simulink model "BoatLibrary"  (Simulink 7.9)
settings: Solver=ode45  StartTime=0.0  StopTime=10.0  RelTol=1e-3
values from neighbouring files (symbols this model uses):
  C = C0    [Minimizer.m]    (also in parameters2.m = [1 0 0 0 0 0;0 0 1 0 0 0;0 0 0 0 1 0]; parameters3.m = [1 0 0 0 0 0;0 0 1 0 0 0;0 0 0 0 1 0])
  fw = 4    [parameters2.m]    (also in parameters3.m)
  I = 1/12*M*((2*rx1)^2 + (2*ry1)^2)    (= 7.46230507536)    [BoatController.m]    (also in boatDynamics.m; parameters2.m = 20; parameters3.m)
  K = [1000 1000 1000 10 10 1 1]    [parameters3.m]
  kr = 2    [parameters2.m]    (also in parameters3.m)
  M = 80*lbtokg    (= 36.28736)    [BoatController.m]    (also in parameters2.m = 10; parameters3.m)
  rx1 = -12*intom    (= -0.3048)    [BoatController.m]    (also in boatDynamics.m; costfunction.m; parameters3.m)
  rx2 = 12*intom    (= 0.3048)    [BoatController.m]    (also in boatDynamics.m; costfunction.m; parameters3.m)
  ry1 = -69*intom/2 + 6*intom    (= -0.7239)    [BoatController.m]    (also in boatDynamics.m; costfunction.m; parameters3.m)
  ry2 = ry1    (= -0.7239)    [BoatController.m]    (also in boatDynamics.m; costfunction.m; parameters3.m)
libraries: simulink x3
settings Model: Creator=Darsan  LastModifiedBy=Darsan

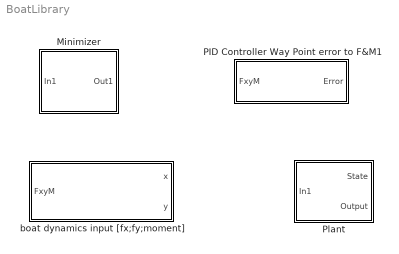
== system BoatLibrary ==
  Minimizer : Subsystem  mask{rx1=rx1, rx2=rx2, ry1=ry1, ry2=ry2, C=K}
      mask prompts: C "Performance Gain"
  PID Controller Way Point error to F&M1 : Subsystem
  Plant : Subsystem  mask{rx1=rx1, rx2=rx2, ry1=ry1, ry2=ry2, M=M, I=I, C=C}
  boat dynamics input [fx;fy;moment] : Subsystem  mask{M=M, I=I, fw=fw, kr=kr, C=C}
      mask prompts: M "Mass"; I "Inert"; fw "Water Friction"; kr "Rotational water Friction"; C "Output Matrix"

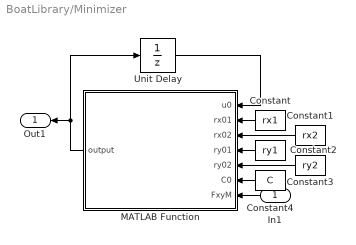
== system BoatLibrary/Minimizer ==
  In1 : Inport
  Constant : Constant  Value=rx1
  Constant1 : Constant  Value=rx2
  Constant2 : Constant  Value=ry1
  Constant3 : Constant  Value=ry2
  Constant4 : Constant  Value=C
  MATLAB Function : MATLAB Function  TreatAsAtomicUnit=on
  Unit Delay : UnitDelay  SampleTime=-1
  Out1 : Outport
  wires:
  In1/1 -> MATLAB Function/7(FxyM)
  MATLAB Function/1(output) -> Out1/1, Unit Delay/1
  Unit Delay/1 -> MATLAB Function/1(u0)
  Constant4/1 -> MATLAB Function/6(C0)
  Constant3/1 -> MATLAB Function/5(ry02)
  Constant2/1 -> MATLAB Function/4(ry01)
  Constant1/1 -> MATLAB Function/3(rx02)
  Constant/1 -> MATLAB Function/2(rx01)

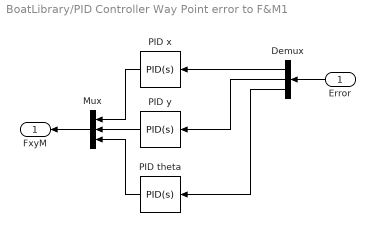
== system BoatLibrary/PID Controller Way Point error to F&M1 ==
  Error : Inport
  Demux : Demux  Outputs=3
  Mux : Mux  Inputs=3
  PID theta : simulink/Continuous/PID Controller  Controller=PID  TimeDomain=Continuous-time  SampleTime=1  IntegratorMethod=Forward Euler  FilterMethod=Forward Euler  Form=Parallel  P=-52.7411095906827  I=-178.448916818041  D=5.47077070641916  N=9.64052643054454  InitialConditionSource=internal  InitialConditionForIntegrator=0  InitialConditionForFilter=0  ExternalReset=none  LimitOutput=off  UpperSaturationLimit=inf  LowerSaturationLimit=-inf  LinearizeAsGain=off  AntiWindupMode=none  Kb=1  TrackingMode=off  Kt=1  PParamMin=[]  PParamMax=[]  IParamMin=[]  IParamMax=[]  DParamMin=[]  DParamMax=[]  NParamMin=[]  NParamMax=[]  KbParamMin=[]  KbParamMax=[]  KtParamMin=[]  KtParamMax=[]  POutMin=[]  POutMax=[]  IOutMin=[]  IOutMax=[]  DOutMin=[]  DOutMax=[]  NOutMin=[]  NOutMax=[]  KbOutMin=[]  KbOutMax=[]  KtOutMin=[]  KtOutMax=[]  IntegratorOutMin=[]  IntegratorOutMax=[]  FilterOutMin=[]  FilterOutMax=[]  SumOutMin=[]  SumOutMax=[]  SumI1OutMin=[]  SumI1OutMax=[]  SumI2OutMin=[]  SumI2OutMax=[]  SumI3OutMin=[]  SumI3OutMax=[]  SumDOutMin=[]  SumDOutMax=[]  SaturationOutMin=[]  SaturationOutMax=[]  IntegratorContinuousStateAttributes=''  IntegratorStateMustResolveToSignalObject=off  IntegratorRTWStateStorageClass=Auto  FilterContinuousStateAttributes=''  FilterStateMustResolveToSignalObject=off  FilterRTWStateStorageClass=Auto
  PID x : simulink/Continuous/PID Controller  Controller=PID  TimeDomain=Continuous-time  SampleTime=1  IntegratorMethod=Forward Euler  FilterMethod=Forward Euler  Form=Parallel  P=-52.7411095906827  I=-356.897833636081  D=2.73538535320958  N=19.2810528610891  InitialConditionSource=internal  InitialConditionForIntegrator=0  InitialConditionForFilter=0  ExternalReset=none  LimitOutput=off  UpperSaturationLimit=inf  LowerSaturationLimit=-inf  LinearizeAsGain=off  AntiWindupMode=none  Kb=1  TrackingMode=off  Kt=1  PParamMin=[]  PParamMax=[]  IParamMin=[]  IParamMax=[]  DParamMin=[]  DParamMax=[]  NParamMin=[]  NParamMax=[]  KbParamMin=[]  KbParamMax=[]  KtParamMin=[]  KtParamMax=[]  POutMin=[]  POutMax=[]  IOutMin=[]  IOutMax=[]  DOutMin=[]  DOutMax=[]  NOutMin=[]  NOutMax=[]  KbOutMin=[]  KbOutMax=[]  KtOutMin=[]  KtOutMax=[]  IntegratorOutMin=[]  IntegratorOutMax=[]  FilterOutMin=[]  FilterOutMax=[]  SumOutMin=[]  SumOutMax=[]  SumI1OutMin=[]  SumI1OutMax=[]  SumI2OutMin=[]  SumI2OutMax=[]  SumI3OutMin=[]  SumI3OutMax=[]  SumDOutMin=[]  SumDOutMax=[]  SaturationOutMin=[]  SaturationOutMax=[]  IntegratorContinuousStateAttributes=''  IntegratorStateMustResolveToSignalObject=off  IntegratorRTWStateStorageClass=Auto  FilterContinuousStateAttributes=''  FilterStateMustResolveToSignalObject=off  FilterRTWStateStorageClass=Auto
  PID y : simulink/Continuous/PID Controller  Controller=PID  TimeDomain=Continuous-time  SampleTime=1  IntegratorMethod=Forward Euler  FilterMethod=Forward Euler  Form=Parallel  P=-52.7411095906827  I=-356.897833636081  D=2.73538535320958  N=19.2810528610891  InitialConditionSource=internal  InitialConditionForIntegrator=0  InitialConditionForFilter=0  ExternalReset=none  LimitOutput=off  UpperSaturationLimit=inf  LowerSaturationLimit=-inf  LinearizeAsGain=off  AntiWindupMode=none  Kb=1  TrackingMode=off  Kt=1  PParamMin=[]  PParamMax=[]  IParamMin=[]  IParamMax=[]  DParamMin=[]  DParamMax=[]  NParamMin=[]  NParamMax=[]  KbParamMin=[]  KbParamMax=[]  KtParamMin=[]  KtParamMax=[]  POutMin=[]  POutMax=[]  IOutMin=[]  IOutMax=[]  DOutMin=[]  DOutMax=[]  NOutMin=[]  NOutMax=[]  KbOutMin=[]  KbOutMax=[]  KtOutMin=[]  KtOutMax=[]  IntegratorOutMin=[]  IntegratorOutMax=[]  FilterOutMin=[]  FilterOutMax=[]  SumOutMin=[]  SumOutMax=[]  SumI1OutMin=[]  SumI1OutMax=[]  SumI2OutMin=[]  SumI2OutMax=[]  SumI3OutMin=[]  SumI3OutMax=[]  SumDOutMin=[]  SumDOutMax=[]  SaturationOutMin=[]  SaturationOutMax=[]  IntegratorContinuousStateAttributes=''  IntegratorStateMustResolveToSignalObject=off  IntegratorRTWStateStorageClass=Auto  FilterContinuousStateAttributes=''  FilterStateMustResolveToSignalObject=off  FilterRTWStateStorageClass=Auto
  FxyM : Outport
  wires:
  Mux/1 -> FxyM/1
  PID theta/1 -> Mux/3
  PID x/1 -> Mux/1
  PID y/1 -> Mux/2
  Error/1 -> Demux/1
  Demux/3 -> PID theta/1
  Demux/2 -> PID y/1
  Demux/1 -> PID x/1

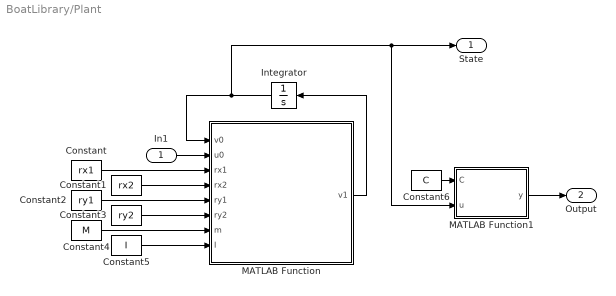
== system BoatLibrary/Plant ==
  In1 : Inport
  Constant : Constant  Value=rx1
  Constant1 : Constant  Value=rx2
  Constant2 : Constant  Value=ry1
  Constant3 : Constant  Value=ry2
  Constant4 : Constant  Value=M
  Constant5 : Constant  Value=I
  Constant6 : Constant  Value=C
  Integrator : Integrator  InitialCondition=[0 0 0 0 0 0]
  MATLAB Function : MATLAB Function  TreatAsAtomicUnit=on
  MATLAB Function1 : MATLAB Function  TreatAsAtomicUnit=on
  State : Outport
  Output : Outport  Port=2
  wires:
  MATLAB Function1/1(y) -> Output/1
  Constant6/1 -> MATLAB Function1/1(C)
  In1/1 -> MATLAB Function/2(u0)
  Integrator/1 -> MATLAB Function1/2(u), State/1, MATLAB Function/1(v0)
  MATLAB Function/1(v1) -> Integrator/1
  Constant5/1 -> MATLAB Function/8(I)
  Constant4/1 -> MATLAB Function/7(m)
  Constant3/1 -> MATLAB Function/6(ry2)
  Constant2/1 -> MATLAB Function/5(ry1)
  Constant1/1 -> MATLAB Function/4(rx2)
  Constant/1 -> MATLAB Function/3(rx1)

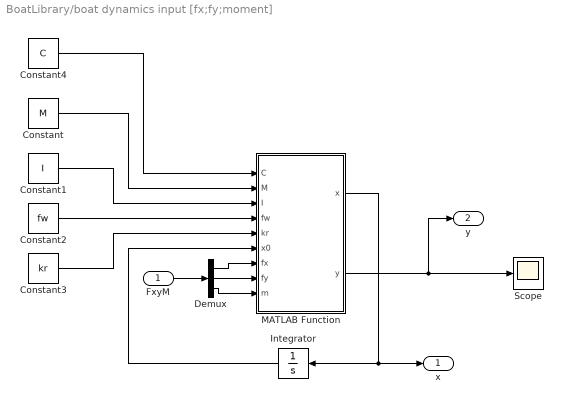
== system BoatLibrary/boat dynamics input [fx;fy;moment] ==
  FxyM : Inport
  Constant : Constant  Value=M
  Constant1 : Constant  Value=I
  Constant2 : Constant  Value=fw
  Constant3 : Constant  Value=kr
  Constant4 : Constant  Value=C
  Demux : Demux  Outputs=3
  Integrator : Integrator  InitialCondition=[0 0 0 0 0 0]
  MATLAB Function : MATLAB Function  TreatAsAtomicUnit=on
  Scope : Scope
  x : Outport
  y : Outport  Port=2
  wires:
  Demux/3 -> MATLAB Function/9(m)
  Demux/2 -> MATLAB Function/8(fy)
  Demux/1 -> MATLAB Function/7(fx)
  FxyM/1 -> Demux/1
  MATLAB Function/1(x) -> x/1, Integrator/1
  Constant4/1 -> MATLAB Function/1(C)
  Constant3/1 -> MATLAB Function/5(kr)
  Constant2/1 -> MATLAB Function/4(fw)
  Constant1/1 -> MATLAB Function/3(I)
  Constant/1 -> MATLAB Function/2(M)
  Integrator/1 -> MATLAB Function/6(x0)
  MATLAB Function/2(y) -> y/1, Scope/1

== matlab function Plant/MATLAB Function ==
  data: v0 input double; v1 output double; u0 input double; rx1 input double; rx2 input double; ry1 input double; ry2 input double; m input double; I input double
function v1   = boatDynamics(v0, u0, rx1, rx2, ry1, ry2, m, I)

    % %%%%%%%%%%%%%%%%%%%%%%%%%%%%%%%%%%%%%%%%%%%% %
    %    v = [x...          %    u = [theta1...    %
    %        x_dot...       %        f1...         %
    %        y...           %        theta2...     %
    %        y_dot...       %        f2]           %
    %        theta...       %                      %
    %        theta_dot];    %                      %
    % %%%%%%%%%%%%%%%%%%%%%%%%%%%%%%%%%%%%%%%%%%%% %
    
    v11 = v0(2);
    v12 = -u0(2)/m*sind(u0(1)+v0(5)) - u0(4)/m*sind(u0(3)+v0(5)) - 0*5*v0(1);
    v13 = v0(4);
    v14 = u0(2)/m*cosd(u0(1)+v0(5)) + u0(4)/m*cosd(u0(3)+v0(5)) - 0*2*v0(3);
    v15 = v0(6);
    v16 = rx1/I*u0(2)*cosd(u0(1)) + ry1/I*u0(2)*sind(u0(1)) + rx2/I*u0(4)*cosd(u0(3)) + ry2/I*u0(4)*sind(u0(3)) - 0*9*v0(5);
   
    v1 = [v11;v12;v13;v14;v15;v16];
    
    
end

== matlab function boat dynamics input [fx;fy;moment]/MATLAB Function ==
  data: C input double; x output double; M input double; I input double; fw input double; kr input double; x0 input double; fx input double; y output double; fy input double; m input double
function [x,y] = systemstep(C,M,I,fw,kr,x0,fx,fy,m)

   % status vector y=[x;x_dot;y;_y_dot;theta;theta_dot]
   % forces u=[fx;fy;m]
   % contant parameters {mass; rotational inertia; friction coefficients }
   
   x1 = x0(2);
   x2 = fx/M - x0(2)*fw;
   x3 = x0(4);
   x4 = fy/M - x0(4)*fw;
   x5 = x0(6);
   x6 = m/I - x0(6)*kr;

   x=[x1;x2;x3;x4;x5;x6];
   
   y = C*x;

== matlab function Minimizer/MATLAB Function ==
  data: u0 input double; output output double; rx01 input double; rx02 input double; ry01 input double; ry02 input double; C0 input double; FxyM input double
function output = Minimizer(u0, rx01, rx02, ry01, ry02, C0, FxyM)

% global rx1 rx2 ry1 ry2 C;
% global Fxref Fyref Mref;

rx1 = rx01; rx2 = rx02;
ry1 = ry01; ry2 = ry02;

C = C0;

Fxref = FxyM(1); Fyref = FxyM(2); Mref  = FxyM(3);
u1 = u0;

    for k = 1:3
        h = getDirection(u1, u0, Fxref, Fyref, Mref, rx1, rx2, ry1, ry2, C);
        alpha = getStepSize(u1, u0, h, Fxref, Fyref, Mref, rx1, rx2, ry1, ry2, C);
        u1 = u1 + alpha*h;
    end
    
    output = u1;

end

function output = getStepSize(input, preinput, h, Fxref, Fyref, Mref, rx1, rx2, ry1, ry2, C)

%     global Fxref Fyref Mref;

    alpha = 1;
    
    u0 = input;
    u1 = input + alpha*h;
    
    v0 = costFunction( u0, preinput, Fxref, Fyref, Mref, rx1, rx2, ry1, ry2, C );
    v1 = costFunction( u1, preinput, Fxref, Fyref, Mref, rx1, rx2, ry1, ry2, C );

    while v1 < v0
        alpha = alpha + 1;
        u1 = input + alpha*h;
        v0 = v1;
        v1 = costFunction( u1, preinput, Fxref, Fyref, Mref, rx1, rx2, ry1, ry2, C );
    end

    while v1 > v0 && alpha > 0
        alpha = alpha - 0.1;
        u1 = input + alpha*h;
        v0 = v1;
        v1 = costFunction( u1, preinput, Fxref, Fyref, Mref, rx1, rx2, ry1, ry2, C );
    end

    output = alpha;

end

function output = costFunction(input, preinput, Fxref, Fyref, Mref, rx1, rx2, ry1, ry2, C)

% global rx1 rx2 ry1 ry2 C;
% global Fxref Fyref Mref;

    theta1  = input(1);
    f1      = input(2);
    theta2  = input(3);
    f2      = input(4);
    
    pretheta1   = preinput(1);
    pretheta2   = preinput(3);

    Fx = f1*sin(theta1) + f2*sin(theta2);
    Fy = f1*cos(theta1) + f2*cos(theta2);
    M = rx1*f1*cos(theta1) - ry1*f1*sin(theta1) + rx2*f2*cos(theta2)...
        - ry2*f2*sin(theta2);

    output = C(1)*(Fx-Fxref)^2 +...
        C(2)*(Fy-Fyref)^2 +...
        C(3)*(M-Mref)^2  +...
        C(4)*f1^2 +...
        C(5)*f2^2 +...
        C(6)*(theta1 - pretheta1)^2 +...
        C(7)*(theta2 - pretheta2)^2;

end

function output = getDirection(input, preinput, Fxref, Fyref, Mref, rx1, rx2, ry1, ry2, C)

hsd = SteepestDescent(input, preinput, Fxref, Fyref, Mref, rx1, rx2, ry1, ry2, C);
hn = Newtons(input, Fxref, Fyref, Mref, rx1, rx2, ry1, ry2, C);

output = zeros(4,1);

    for i = 1:length(hn)

        if sign(hn(i)) > 0
            output(i) = hn(i);
        else
            output(i) = hsd(i);
        end
    end
end

function output = SteepestDescent(input, preinput, Fxref, Fyref, Mref, rx1, rx2, ry1, ry2, C)

% global rx1 rx2 ry1 ry2 C;
% global Fxref Fyref Mref;

theta1  = input(1);
f1      = input(2);
theta2  = input(3);
f2      = input(4);

pretheta1   = preinput(1);
pretheta2   = preinput(3);

dVdtheta1 = 2*C(3)*(f1*ry1*cos(theta1) + f1*rx1*sin(theta1))*(Mref ...
    - f1*rx1*cos(theta1) - f2*rx2*cos(theta2) + f1*ry1*sin(theta1) ...
    + f2*ry2*sin(theta2)) - C(6)*(2*pretheta1 - 2*theta1) ...
    - 2*C(2)*f1*sin(theta1)*(f1*cos(theta1) - Fyref + f2*cos(theta2)) ...
    + 2*C(1)*f1*cos(theta1)*(f1*sin(theta1) - Fxref + f2*sin(theta2));

dVdf1 = 2*C(4)*f1 - 2*C(3)*(rx1*cos(theta1) - ry1*sin(theta1))*(Mref ...
    - f1*rx1*cos(theta1) - f2*rx2*cos(theta2) + f1*ry1*sin(theta1) ...
    + f2*ry2*sin(theta2)) + 2*C(2)*cos(theta1)*(f1*cos(theta1) - Fyref ...
    + f2*cos(theta2)) + 2*C(1)*sin(theta1)*(f1*sin(theta1) - Fxref ...
    + f2*sin(theta2));

dVdtheta2 = 2*C(3)*(f2*ry2*cos(theta2) + f2*rx2*sin(theta2))*(Mref ...
    - f1*rx1*cos(theta1) - f2*rx2*cos(theta2) + f1*ry1*sin(theta1) ...
    + f2*ry2*sin(theta2)) - C(7)*(2*pretheta2 - 2*theta2) ...
    - 2*C(2)*f2*sin(theta2)*(f1*cos(theta1) - Fyref + f2*cos(theta2)) ...
    + 2*C(1)*f2*cos(theta2)*(f1*sin(theta1) - Fxref + f2*sin(theta2));

dVdf2 = 2*C(5)*f2 - 2*C(3)*(rx2*cos(theta2) - ry2*sin(theta2))*(Mref ...
    - f1*rx1*cos(theta1) - f2*rx2*cos(theta2) + f1*ry1*sin(theta1) ...
    + f2*ry2*sin(theta2)) + 2*C(2)*cos(theta2)*(f1*cos(theta1) - Fyref ...
    + f2*cos(theta2)) + 2*C(1)*sin(theta2)*(f1*sin(theta1) - Fxref ...
    + f2*sin(theta2));

output = -[dVdtheta1; dVdf1; dVdtheta2; dVdf2];

end

function output = Newtons(input, Fxref, Fyref, Mref, rx1, rx2, ry1, ry2, C)
% global rx1 rx2 ry1 ry2 C;
% global Fxref Fyref Mref;

theta1  = input(1);
f1      = input(2);
theta2  = input(3);
f2      = input(4);

ddVddtheta1 = 2*C(6) + 2*C(3)*(f1*ry1*cos(theta1) + f1*rx1*sin(theta1))^2 ...
    + 2*C(3)*(f1*rx1*cos(theta1) - f1*ry1*sin(theta1))*(Mref ...
    - f1*rx1*cos(theta1) - f2*rx2*cos(theta2) + f1*ry1*sin(theta1) ...
    + f2*ry2*sin(theta2)) + 2*C(1)*f1^2*cos(theta1)^2 ...
    + 2*C(2)*f1^2*sin(theta1)^2 - 2*C(2)*f1*cos(theta1)*(f1*cos(theta1) ...
    - Fyref + f2*cos(theta2)) - 2*C(1)*f1*sin(theta1)*(f1*sin(theta1) ...
    - Fxref + f2*sin(theta2));

ddVddf1 = 2*C(4) + 2*C(3)*(rx1*cos(theta1) - ry1*sin(theta1))^2 ...
    + 2*C(2)*cos(theta1)^2 + 2*C(1)*sin(theta1)^2;

ddVddtheta2 = 2*C(7) + 2*C(3)*(f2*ry2*cos(theta2) + f2*rx2*sin(theta2))^2 ...
    + 2*C(3)*(f2*rx2*cos(theta2) - f2*ry2*sin(theta2))*(Mref ...
    - f1*rx1*cos(theta1) - f2*rx2*cos(theta2) + f1*ry1*sin(theta1) ...
    + f2*ry2*sin(theta2)) + 2*C(1)*f2^2*cos(theta2)^2 ...
    + 2*C(2)*f2^2*sin(theta2)^2 - 2*C(2)*f2*cos(theta2)*(f1*cos(theta1) ...
    - Fyref + f2*cos(theta2)) - 2*C(1)*f2*sin(theta2)*(f1*sin(theta1) ...
    - Fxref + f2*sin(theta2));

ddVddf2 = 2*C(5) + 2*C(3)*(rx2*cos(theta2) - ry2*sin(theta2))^2 ...
    + 2*C(2)*cos(theta2)^2 + 2*C(1)*sin(theta2)^2;
 


output = [ddVddtheta1; ddVddf1; ddVddtheta2; ddVddf2];

end

== matlab function Plant/MATLAB Function1 ==
  data: C input double; u input double; y output double
function y = fcn(C,u)
%#codegen

y = C*u;
